simulink subsystem "Sample_Catmull_Rom_Pos_And_Curve"  (R2023b)
settings: Solver=VariableStepAuto  StartTime=0.0  StopTime=10.0  RelTol=1e-3
undefined symbols (not defined in the file): Spline_Num_Samples
settings Model: Creator=FIRSTMentor  LastModifiedBy=ander

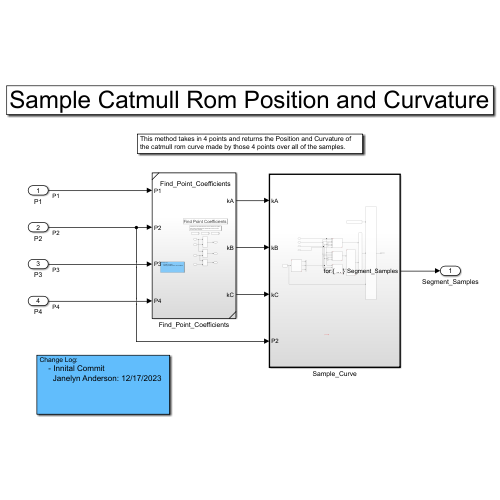
[thumbnail: Simulink's stored preview of the top-level diagram]
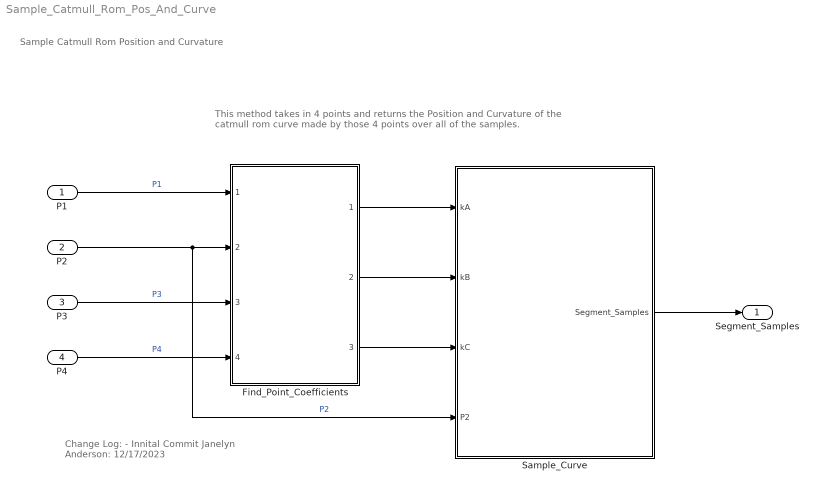
== system Sample_Catmull_Rom_Pos_And_Curve ==
  note: Sample Catmull Rom Position and Curvature
  note: This method takes in 4 points and returns the Position and Curvature of the catmull rom curve made by those 4 points over all of the samples.
  note: Change Log:
      | - Innital Commit
      | Janelyn Anderson: 12/17/2023
  P1 : Inport  PortDimensions=[1 2]
  P2 : Inport  Port=2  PortDimensions=[1 2]
  P3 : Inport  Port=3  PortDimensions=[1 2]
  P4 : Inport  Port=4  PortDimensions=[1 2]
  Find_Point_Coefficients : Subsystem  ReferencedSubsystem=Find_Point_Coefficients
  Sample_Curve : Subsystem  TreatAsAtomicUnit=on
  Segment_Samples : Outport
  wires:
  Find_Point_Coefficients/3 -> Sample_Curve/3(kC)
  Sample_Curve/1(Segment_Samples) -> Segment_Samples/1
  P1/1 -> Find_Point_Coefficients/1  "P1"
  Find_Point_Coefficients/1 -> Sample_Curve/1(kA)
  P4/1 -> Find_Point_Coefficients/4  "P4"
  Find_Point_Coefficients/2 -> Sample_Curve/2(kB)
  P2/1 -> Sample_Curve/4(P2), Find_Point_Coefficients/2  "P2"
  P3/1 -> Find_Point_Coefficients/3  "P3"

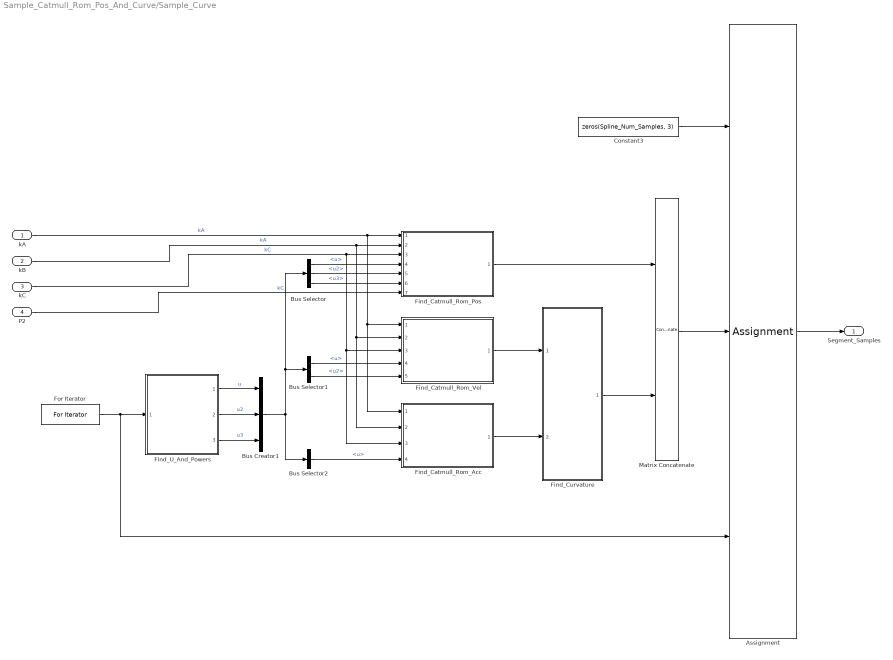
== system Sample_Catmull_Rom_Pos_And_Curve/Sample_Curve ==
  kA : Inport  PortDimensions=[1 2]
  kB : Inport  Port=2  PortDimensions=[1 2]
  kC : Inport  Port=3  PortDimensions=[1 2]
  P2 : Inport  Port=4  PortDimensions=[1 2]
  Assignment : Assignment  NumberOfDimensions=2  DiagnosticForDimensions=Warning  IndexOptions=Index vector (port),Assign all  Indices=1,1  OutputSizes=1,1
  Bus Creator1 : BusCreator  Inputs=3
  Bus Selector : BusSelector  OutputSignals=u,u2,u3
  Bus Selector1 : BusSelector  OutputSignals=u,u2
  Bus Selector2 : BusSelector  OutputSignals=u
  Constant3 : Constant  Value=zeros(Spline_Num_Samples, 3)
  Find_Catmull_Rom_Acc : Subsystem  ReferencedSubsystem=Find_Catmull_Rom_Acc
  Find_Catmull_Rom_Pos : Subsystem  ReferencedSubsystem=Find_Catmull_Rom_Pos
  Find_Catmull_Rom_Vel : Subsystem  ReferencedSubsystem=Find_Catmull_Rom_Vel
  Find_Curvature : Subsystem  ReferencedSubsystem=Find_Curvature
  Find_U_And_Powers : Subsystem  ReferencedSubsystem=Find_U_And_Powers
  For Iterator : ForIterator  IterationLimit=Spline_Num_Samples
  Matrix Concatenate : Concatenate  Mode=Multidimensional array  ConcatenateDimension=2
  Segment_Samples : Outport
  wires:
  Find_U_And_Powers/3 -> Bus Creator1/3  "u3"
  Find_U_And_Powers/1 -> Bus Creator1/1  "u"
  Find_U_And_Powers/2 -> Bus Creator1/2  "u2"
  P2/1 -> Find_Catmull_Rom_Pos/7  "kC"
  Matrix Concatenate/1 -> Assignment/2
  Find_Catmull_Rom_Pos/1 -> Matrix Concatenate/1
  Find_Catmull_Rom_Acc/1 -> Find_Curvature/2
  Find_Catmull_Rom_Vel/1 -> Find_Curvature/1
  kC/1 -> Find_Catmull_Rom_Vel/3, Find_Catmull_Rom_Acc/3, Find_Catmull_Rom_Pos/3  "kC"
  kB/1 -> Find_Catmull_Rom_Pos/2, Find_Catmull_Rom_Vel/2, Find_Catmull_Rom_Acc/2  "kA"
  kA/1 -> Find_Catmull_Rom_Pos/1, Find_Catmull_Rom_Vel/1, Find_Catmull_Rom_Acc/1  "kA"
  Bus Selector2/1 -> Find_Catmull_Rom_Acc/4  "<u>"
  Bus Selector1/2 -> Find_Catmull_Rom_Vel/5  "<u2>"
  Bus Selector1/1 -> Find_Catmull_Rom_Vel/4  "<u>"
  Bus Selector/2 -> Find_Catmull_Rom_Pos/5  "<u2>"
  Bus Selector/3 -> Find_Catmull_Rom_Pos/6  "<u3>"
  Bus Selector/1 -> Find_Catmull_Rom_Pos/4  "<u>"
  Bus Creator1/1 -> Bus Selector1/1, Bus Selector/1, Bus Selector2/1
  Assignment/1 -> Segment_Samples/1
  Constant3/1 -> Assignment/1
  For Iterator/1 -> Find_U_And_Powers/1, Assignment/3
  Find_Curvature/1 -> Matrix Concatenate/2
